simulink model "quadrotor_PID_Hinf_Synthesis_decentralized_simulink"  (R2023b)
settings: Solver=ode4  StartTime=0.0  StopTime=10  FixedStep=0.001  RelTol=1e-3
values from neighbouring files (symbols this model uses):
  A_x_in = [0 1; 0 0]    [quadrotor_PID_Hinf_Backstepping_decentralized.m]    (also in quadrotor_PID_Hinf_Synthesis_decentralized.m; quadrotor_PID_LQR_decentralized.m)
  A_x_out = [0 1; 0 0]    [quadrotor_PID_Hinf_Backstepping_decentralized.m]    (also in quadrotor_PID_Hinf_Synthesis_decentralized.m; quadrotor_PID_LQR_decentralized.m)
  A_y_in = [0 1; 0 0]    [quadrotor_PID_Hinf_Backstepping_decentralized.m]    (also in quadrotor_PID_Hinf_Synthesis_decentralized.m; quadrotor_PID_LQR_decentralized.m)
  A_y_out = [0 1; 0 0]    [quadrotor_PID_Hinf_Backstepping_decentralized.m]    (also in quadrotor_PID_Hinf_Synthesis_decentralized.m; quadrotor_PID_LQR_decentralized.m)
  Ayaw = [0 1; 0 0]    [quadrotor_PID_Hinf_Backstepping_decentralized.m]    (also in quadrotor_PID_Hinf_Synthesis_decentralized.m; quadrotor_PID_LQR_decentralized.m)
  Az = [0 1; 0 0]    [quadrotor_PID_Hinf_Backstepping_decentralized.m]    (also in quadrotor_PID_Hinf_Synthesis_decentralized.m; quadrotor_PID_LQR_decentralized.m)
  B_x_in = [0; 1/Iy]    [quadrotor_PID_Hinf_Backstepping_decentralized.m]    (also in quadrotor_PID_Hinf_Synthesis_decentralized.m; quadrotor_PID_LQR_decentralized.m)
  B_x_out = [0; g]    [quadrotor_PID_Hinf_Backstepping_decentralized.m]    (also in quadrotor_PID_Hinf_Synthesis_decentralized.m; quadrotor_PID_LQR_decentralized.m)
  B_y_in = [0; 1/Ix]    [quadrotor_PID_Hinf_Backstepping_decentralized.m]    (also in quadrotor_PID_Hinf_Synthesis_decentralized.m; quadrotor_PID_LQR_decentralized.m)
  B_y_out = [0; -g]    [quadrotor_PID_Hinf_Backstepping_decentralized.m]    (also in quadrotor_PID_Hinf_Synthesis_decentralized.m; quadrotor_PID_LQR_decentralized.m)
  Byaw = [0; 1/Iz]    [quadrotor_PID_Hinf_Backstepping_decentralized.m]    (also in quadrotor_PID_Hinf_Synthesis_decentralized.m; quadrotor_PID_LQR_decentralized.m)
  Bz = [0; 1/m]    [quadrotor_PID_Hinf_Backstepping_decentralized.m]    (also in quadrotor_PID_Hinf_Synthesis_decentralized.m; quadrotor_PID_LQR_decentralized.m)
  C_x_in = [1 0]    [quadrotor_PID_Hinf_Backstepping_decentralized.m]    (also in quadrotor_PID_Hinf_Synthesis_decentralized.m; quadrotor_PID_LQR_decentralized.m)
  C_x_out = [1 0]    [quadrotor_PID_Hinf_Backstepping_decentralized.m]    (also in quadrotor_PID_Hinf_Synthesis_decentralized.m; quadrotor_PID_LQR_decentralized.m)
  C_y_in = [1 0]    [quadrotor_PID_Hinf_Backstepping_decentralized.m]    (also in quadrotor_PID_Hinf_Synthesis_decentralized.m; quadrotor_PID_LQR_decentralized.m)
  C_y_out = [1 0]    [quadrotor_PID_Hinf_Backstepping_decentralized.m]    (also in quadrotor_PID_Hinf_Synthesis_decentralized.m; quadrotor_PID_LQR_decentralized.m)
  Cyaw = [1 0]    [quadrotor_PID_Hinf_Backstepping_decentralized.m]    (also in quadrotor_PID_Hinf_Synthesis_decentralized.m; quadrotor_PID_LQR_decentralized.m)
  Cz = [1 0]    [quadrotor_PID_Hinf_Backstepping_decentralized.m]    (also in quadrotor_PID_Hinf_Synthesis_decentralized.m; quadrotor_PID_LQR_decentralized.m)
undefined symbols (not defined in the file or in its folder): Kd_x_in, Kd_x_out, Kd_y_in, Kd_y_out, Kd_yaw, Kd_z, Ki_x_in, Ki_x_out, Ki_y_in, Ki_y_out, Ki_yaw, Ki_z, Kp_x_in, Kp_x_out, Kp_y_in, Kp_y_out, Kp_yaw, Kp_z
libraries: dspsrcs4 x3, simulink x2
settings Model: Creator=izmah  LastModifiedBy=izmah

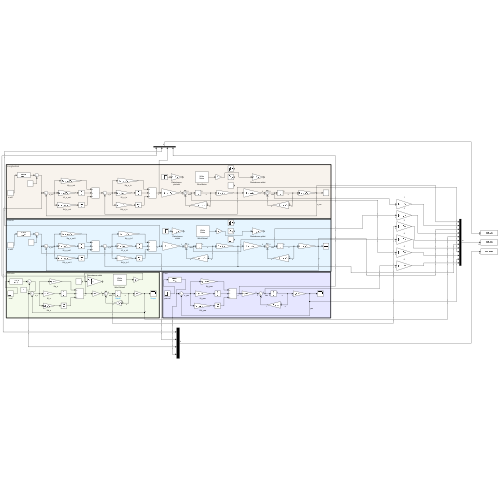
[thumbnail: Simulink's stored preview of the top-level diagram]
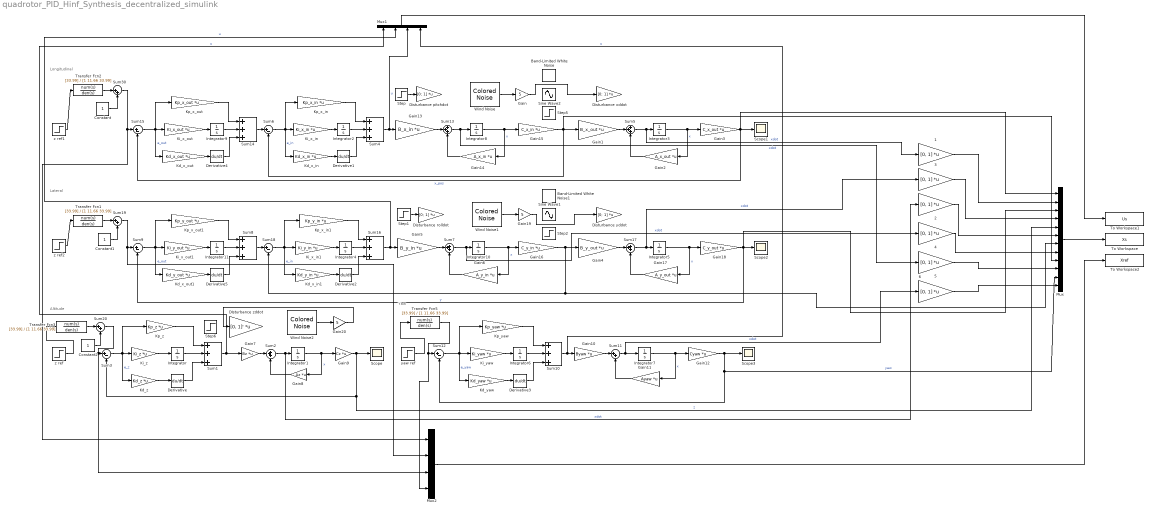
== system quadrotor_PID_Hinf_Synthesis_decentralized_simulink ==
  note: Longitudinal
  note: Lateral
  note: Altitude
  note: Yaw
  {1..6} (6 alike) : Gain  Gain=[0, 1]  Multiplication=Matrix(K*u)
  Band-Limited White Noise : simulink/Sources/Band-Limited White Noise  Cov=[0.5]  Ts=0.1  seed=[23341]
  Band-Limited White Noise1 : simulink/Sources/Band-Limited White Noise  Cov=[0.5]  Ts=0.1  seed=[23341]
  Constant : Constant
  Constant1 : Constant
  Constant2 : Constant
  DIsturbance zddot : Gain  Gain=[0, 1]'  Multiplication=Matrix(K*u)
  Derivative{,1..5} (6 alike) : Derivative
  Disturbance pitchdot : Gain  Gain=[0; 1]  Multiplication=Matrix(K*u)
  Disturbance rolldot : Gain  Gain=[0; 1]  Multiplication=Matrix(K*u)
  Disturbance xddot : Gain  Gain=[0; 1]  Multiplication=Matrix(K*u)
  Disturbance yddot : Gain  Gain=[0; 1]  Multiplication=Matrix(K*u)
  Gain : Gain  Gain=5
  Gain1 : Gain  Gain=B_x_out  Multiplication=Matrix(K*u)
  Gain10 : Gain  Gain=Byaw  Multiplication=Matrix(K*u)
  Gain11 : Gain  Gain=Ayaw  Multiplication=Matrix(K*u)
  Gain12 : Gain  Gain=Cyaw  Multiplication=Matrix(K*u)
  Gain13 : Gain  Gain=B_x_in  Multiplication=Matrix(K*u)
  Gain14 : Gain  Gain=A_x_in  Multiplication=Matrix(K*u)
  Gain15 : Gain  Gain=C_x_in  Multiplication=Matrix(K*u)
  Gain16 : Gain  Gain=C_y_in  Multiplication=Matrix(K*u)
  Gain17 : Gain  Gain=A_y_out  Multiplication=Matrix(K*u)
  Gain18 : Gain  Gain=C_y_out  Multiplication=Matrix(K*u)
  Gain19 : Gain  Gain=5
  Gain2 : Gain  Gain=A_x_out  Multiplication=Matrix(K*u)
  Gain20 : Gain  Gain=5
  Gain3 : Gain  Gain=C_x_out  Multiplication=Matrix(K*u)
  Gain4 : Gain  Gain=B_y_out  Multiplication=Matrix(K*u)
  Gain5 : Gain  Gain=B_y_in  Multiplication=Matrix(K*u)
  Gain6 : Gain  Gain=A_y_in  Multiplication=Matrix(K*u)
  Gain7 : Gain  Gain=Bz  Multiplication=Matrix(K*u)
  Gain8 : Gain  Gain=Az  Multiplication=Matrix(K*u)
  Gain9 : Gain  Gain=Cz  Multiplication=Matrix(K*u)
  Integrator{,2,4,6..11} (9 alike) : Integrator
  Integrator1 : Integrator  InitialCondition=[1;0]
  Integrator3 : Integrator  InitialCondition=[1;0]
  Integrator5 : Integrator  InitialCondition=[1;0]
  Kd_x_in : Gain  Gain=Kd_x_in  Multiplication=Matrix(K*u)
  Kd_x_in1 : Gain  Gain=Kd_y_in  Multiplication=Matrix(K*u)
  Kd_x_out : Gain  Gain=Kd_x_out  Multiplication=Matrix(K*u)
  Kd_x_out1 : Gain  Gain=Kd_y_out  Multiplication=Matrix(K*u)
  Kd_yaw : Gain  Gain=Kd_yaw  Multiplication=Matrix(K*u)
  Kd_z : Gain  Gain=Kd_z  Multiplication=Matrix(K*u)
  Ki_x_in : Gain  Gain=Ki_x_in  Multiplication=Matrix(K*u)
  Ki_x_in1 : Gain  Gain=Ki_y_in  Multiplication=Matrix(K*u)
  Ki_x_out : Gain  Gain=Ki_x_out  Multiplication=Matrix(K*u)
  Ki_x_out1 : Gain  Gain=Ki_y_out  Multiplication=Matrix(K*u)
  Ki_yaw : Gain  Gain=Ki_yaw  Multiplication=Matrix(K*u)
  Ki_z : Gain  Gain=Ki_z  Multiplication=Matrix(K*u)
  Kp_x_in : Gain  Gain=Kp_x_in  Multiplication=Matrix(K*u)
  Kp_x_in1 : Gain  Gain=Kp_y_in  Multiplication=Matrix(K*u)
  Kp_x_out : Gain  Gain=Kp_x_out  Multiplication=Matrix(K*u)
  Kp_x_out1 : Gain  Gain=Kp_y_out  Multiplication=Matrix(K*u)
  Kp_yaw : Gain  Gain=Kp_yaw  Multiplication=Matrix(K*u)
  Kp_z : Gain  Gain=Kp_z  Multiplication=Matrix(K*u)
  Mux : Mux  Inputs=12
  Mux1 : Mux
  Mux2 : Mux
  Scope{,1..3} (4 alike) : Scope
  Sine Wave1 : Sin  Frequency=5  SampleTime=0
  Sine Wave2 : Sin  Frequency=5  SampleTime=0
  Step : Step  SampleTime=0
  Step1 : Step  SampleTime=0
  Step2 : Step  Time=0  Before=1  SampleTime=0
  Step5 : Step  Time=0  Before=1  SampleTime=0
  Step6 : Step  Time=5  SampleTime=0
  Sum{1..2,4..5,7..8,10,13..14,16..17} (11 alike) : Sum  Inputs=+++
  Sum{11,19..20,30} (4 alike) : Sum  Inputs=|++
  Sum{3,6,9,12,15,18} (6 alike) : Sum  Inputs=|+-
  To Workspace : ToWorkspace  VariableName=Xs  SampleTime=-1
  To Workspace1 : ToWorkspace  VariableName=Us  SampleTime=-1
  To Workspace2 : ToWorkspace  VariableName=Xref  SampleTime=-1
  Transfer Fcn{1..3,5} (4 alike) : TransferFcn  Numerator=[33.99]  Denominator=[1 11.66 33.99]
  Wind Noise : dspsrcs4/Colored Noise  Color=white  InverseFrequencyPower=1  BoundedOutput=off  NumChannels=1  OutputDataType=double  SamplesPerFrame=1  SampleTime=0.01  RandomStream=mt19937ar with seed  Seed=67  SimulateUsing=Interpreted execution
  Wind Noise1 : dspsrcs4/Colored Noise  Color=white  InverseFrequencyPower=1  BoundedOutput=off  NumChannels=1  OutputDataType=double  SamplesPerFrame=1  SampleTime=0.01  RandomStream=mt19937ar with seed  Seed=67  SimulateUsing=Interpreted execution
  Wind Noise2 : dspsrcs4/Colored Noise  Color=white  InverseFrequencyPower=1  BoundedOutput=off  NumChannels=1  OutputDataType=double  SamplesPerFrame=1  SampleTime=0.01  RandomStream=mt19937ar with seed  Seed=67  SimulateUsing=Interpreted execution
  yaw ref : Step  Time=0.001  After=deg2rad(10)  SampleTime=0
  z ref : Step  Time=0.001  SampleTime=0
  z ref1 : Step  Time=0.001  SampleTime=0
  z ref2 : Step  Time=0.001  SampleTime=0
  wires:
  Integrator/1 -> Sum1/2
  Kd_yaw/1 -> Derivative3/1
  Kd_x_out/1 -> Derivative4/1
  Kd_x_in/1 -> Derivative1/1
  Gain9/1 -> Mux/5, Sum3/2, Scope/1  "z"
  Kp_yaw/1 -> Sum10/1
  Sum17/1 -> 3/1, Integrator5/1  "xdot"
  Ki_z/1 -> Integrator/1
  Sum1/1 -> Gain7/1, Mux1/1  "u"
  Gain16/1 -> Mux/7, Sum18/2, Gain4/1
  z ref1/1 -> Transfer Fcn2/1
  Integrator8/1 -> Gain15/1, Gain14/1  "x"
  Derivative/1 -> Sum1/3
  Integrator6/1 -> Sum10/2
  Integrator7/1 -> Gain11/1, Gain12/1  "x"
  Ki_x_in/1 -> Integrator2/1
  Kd_z/1 -> Derivative/1
  Gain10/1 -> Sum11/1
  Sum18/1 -> Kd_x_in1/1, Ki_x_in1/1, Kp_x_in1/1  "e_in"
  Derivative4/1 -> Sum14/3
  Ki_x_in1/1 -> Integrator4/1
  Derivative1/1 -> Sum4/3
  Sum14/1 -> Sum6/1
  Sum6/1 -> Ki_x_in/1, Kp_x_in/1, Kd_x_in/1  "e_in"
  Sum5/1 -> 1/1, Integrator3/1  "xdot"
  Sum7/1 -> 4/1, Integrator10/1  "xdot"
  Sum15/1 -> Ki_x_out/1, Kp_x_out/1, Kd_x_out/1  "e_out"
  Ki_x_out1/1 -> Integrator11/1
  z ref2/1 -> Transfer Fcn1/1
  Sum13/1 -> 5/1, Integrator8/1  "xdot"
  Integrator1/1 -> Gain8/1, Gain9/1  "x"
  Sum11/1 -> 6/1, Integrator7/1  "xdot"
  Sum10/1 -> Mux1/4, Gain10/1  "u"
  Sum12/1 -> Kd_yaw/1, Ki_yaw/1, Kp_yaw/1  "e_yaw"
  Gain11/1 -> Sum11/2
  Kp_x_out/1 -> Sum14/1
  Integrator11/1 -> Sum8/2
  Kd_x_out1/1 -> Derivative5/1
  Sum9/1 -> Kd_x_out1/1, Ki_x_out1/1, Kp_x_out1/1  "e_out"
  Kd_x_in1/1 -> Derivative2/1
  Integrator3/1 -> Gain3/1, Gain2/1  "x"
  Sum3/1 -> Kd_z/1, Ki_z/1, Kp_z/1  "e_z"
  Ki_x_out/1 -> Integrator9/1
  Kp_z/1 -> Sum1/1
  Integrator10/1 -> Gain6/1, Gain16/1  "x"
  Integrator5/1 -> Gain17/1, Gain18/1  "x"
  Gain15/1 -> Sum6/2, Mux/9, Gain1/1
  Ki_yaw/1 -> Integrator6/1
  Derivative5/1 -> Sum8/3
  Gain3/1 -> Sum15/2, Mux/1, Scope1/1  "x_pos"
  Kp_x_out1/1 -> Sum8/1
  Gain12/1 -> Mux/11, Sum12/2, Scope3/1  "yaw"
  Integrator9/1 -> Sum14/2
  Integrator2/1 -> Sum4/2
  Sum2/1 -> 2/1, Integrator1/1  "xdot"
  Gain18/1 -> Mux/3, Sum9/2, Scope2/1  "y"
  Sum8/1 -> Sum18/1
  Kp_x_in/1 -> Sum4/1
  Sum16/1 -> Mux1/2, Gain5/1  "u"
  Derivative3/1 -> Sum10/3
  Kp_x_in1/1 -> Sum16/1
  Integrator4/1 -> Sum16/2
  Sum4/1 -> Mux1/3, Gain13/1  "u"
  Derivative2/1 -> Sum16/3
  Gain13/1 -> Sum13/2
  Gain14/1 -> Sum13/3
  Gain1/1 -> Sum5/2
  Gain2/1 -> Sum5/3
  Step/1 -> Disturbance pitchdot/1
  Gain/1 -> Disturbance xddot/1
  Step1/1 -> Disturbance rolldot/1
  Gain5/1 -> Sum7/2
  Gain6/1 -> Sum7/3
  Gain4/1 -> Sum17/2
  Gain17/1 -> Sum17/3
  Gain19/1 -> Disturbance yddot/1
  Gain7/1 -> Sum2/2
  Gain8/1 -> Sum2/3
  Sum30/1 -> Mux2/1, Sum15/1
  Sum19/1 -> Mux2/2, Sum9/1
  Wind Noise/1 -> Gain/1
  Wind Noise1/1 -> Gain19/1
  Wind Noise2/1 -> Gain20/1
  Gain20/1 -> DIsturbance zddot/1
  Constant/1 -> Sum30/2
  Transfer Fcn2/1 -> Sum30/1
  Transfer Fcn1/1 -> Sum19/1
  Constant1/1 -> Sum19/2
  Transfer Fcn3/1 -> Sum20/1
  Constant2/1 -> Sum20/2
  z ref/1 -> Transfer Fcn3/1
  Sum20/1 -> Mux2/3, Sum3/1
  yaw ref/1 -> Transfer Fcn5/1
  Transfer Fcn5/1 -> Mux2/4, Sum12/1
  Mux/1 -> To Workspace/1
  Mux1/1 -> To Workspace1/1
  Mux2/1 -> To Workspace2/1
  1/1 -> Mux/2
  3/1 -> Mux/4
  2/1 -> Mux/6
  4/1 -> Mux/8
  5/1 -> Mux/10
  6/1 -> Mux/12
